simulink model "ship_2d_polar"  (R2021b)
settings: Solver=VariableStepAuto  StartTime=0.0  StopTime=10.0  RelTol=1e-3
settings Model: Creator=cirie  LastModifiedBy=cirie

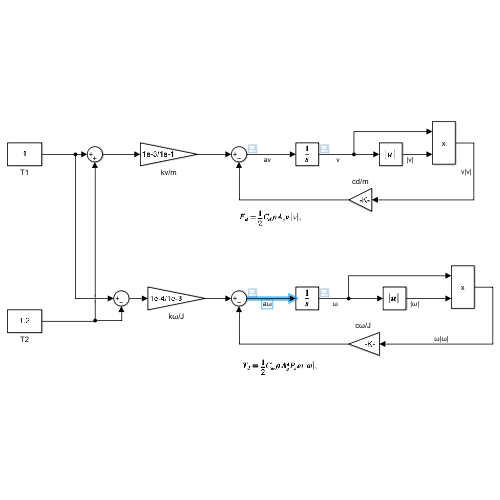
[thumbnail: Simulink's stored preview of the top-level diagram]
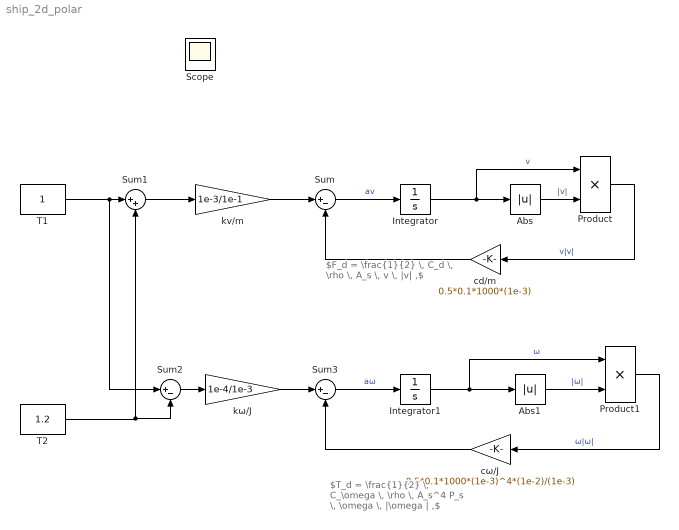
== system ship_2d_polar ==
  note: $F_d = \frac{1}{2} \, C_d \, \rho \, A_s \, v \, |v| ,$
  note: $T_d = \frac{1}{2} \, C_\omega \, \rho \, A_s^4 P_s \, \omega \, |\omega | ,$
  Abs : Abs
  Abs1 : Abs
  Integrator : Integrator  InitialCondition=[0 0]
  Integrator1 : Integrator  InitialCondition=[0 0]
  Product : Product
  Product1 : Product
  Sum : Sum  Inputs=|+-
  Sum1 : Sum  Inputs=|++
  Sum2 : Sum  Inputs=|+-
  Sum3 : Sum  Inputs=|+-
  T1 : Constant
  T2 : Constant  Value=1.2
  cd/m : Gain  Gain=0.5*0.1*1000*(1e-3)
  "cω/J " : Gain  Gain=0.5*0.1*1000*(1e-3)^4*(1e-2)/(1e-3)
  kv/m : Gain  Gain=1e-3/1e-1
  kω/J : Gain  Gain=1e-4/1e-3
  Scope : Scope
  wires:
  Sum/1 -> Integrator/1  "av"
  Integrator/1 -> Product/1, Abs/1  "v"
  Product/1 -> cd/m/1  "v|v|"
  cd/m/1 -> Sum/2
  T1/1 -> Sum1/1, Sum2/1
  T2/1 -> Sum2/2, Sum1/2
  Sum1/1 -> kv/m/1
  Sum2/1 -> kω/J/1
  kv/m/1 -> Sum/1
  kω/J/1 -> Sum3/1
  "cω/J "/1 -> Sum3/2
  Product1/1 -> "cω/J "/1  "ω|ω|"
  Integrator1/1 -> Product1/1, Abs1/1  "ω"
  Sum3/1 -> Integrator1/1  "aω"
  Abs/1 -> Product/2  "|v|"
  Abs1/1 -> Product1/2  "|ω|"
